simulink model "Hysteresis_chart"  (R2020b)
settings: Solver=VariableStepAuto  StartTime=0.0  StopTime=10.0  RelTol=1e-3
settings Model: Creator=Training  LastModifiedBy=Training

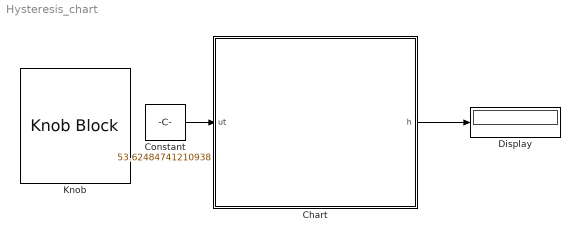
== system Hysteresis_chart ==
  Chart : Stateflow chart  TreatAsAtomicUnit=on
  Constant : Constant  Value=53.62484741210938
  Display : Display
  Knob : KnobBlock
  wires:
  Chart/1(h) -> Display/1
  Constant/1 -> Chart/1(ut)

== stateflow chart Hysteresis_chart/Chart ==
  state Def
  state NoOperation
    entry:
    h=0;
  state HeaterOn
    entry:
    h=1;
  state CoolerOn
    entry:
    h=-1;
  (default) -> Def
  Def -> (junction 11) [order 1]
  Def -> (junction 16) [order 3]
  (junction 11) -> NoOperation : [ut==at]
  (junction 16) -> CoolerOn : [at>ut &&at-ut >= delta]
  Def -> HeaterOn [order 2] : [at<ut &&ut-at >= delta]
  data: at local =23; delta local =2; h output; ut input
